simulink model "quater_car"  (R2025b)
settings: Solver=FixedStepAuto  StartTime=0.0  StopTime=10.0  FixedStep=0.001  RelTol=1e-3
values from neighbouring files (symbols this model uses):
  cs = cs_n(n)    [sim2.m]    (also in sim2_part2.m = 50)
  cs_nolinear = i    [sim2_part2.m]
  ct = 0.01 * 12    (= 0.12)    [sim2.m]    (also in sim2_part2.m)
  ks = 100 * 12    (= 1200)    [sim2.m]    (also in sim2_part2.m)
  kt = 1000 * 12    (= 12000)    [sim2.m]    (also in sim2_part2.m)
  ms = Ws/g    (= 83.9291265154)    [Final_sim.m]    (also in Final_sim_nonlinear.m; sim2.m = 31.0848616724; sim2_part2.m = 31.0848616724)
  mu = 100/32.17    (= 3.10848616724)    [sim2.m]    (also in sim2_part2.m)
  Road_type = 6    [sim2_part2.m]
libraries: dspsrcs4 x1
settings Model: Creator=elijah  LastModifiedBy=elijah

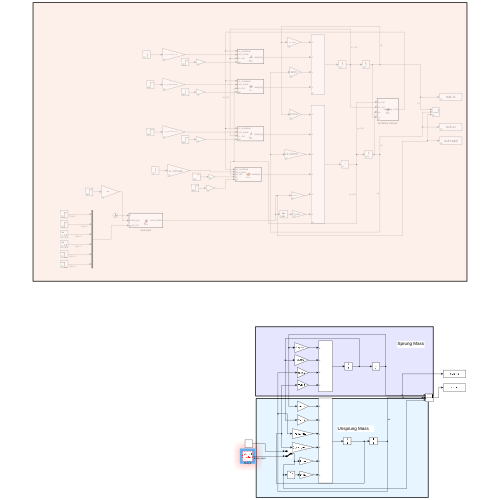
[thumbnail: Simulink's stored preview of the top-level diagram]
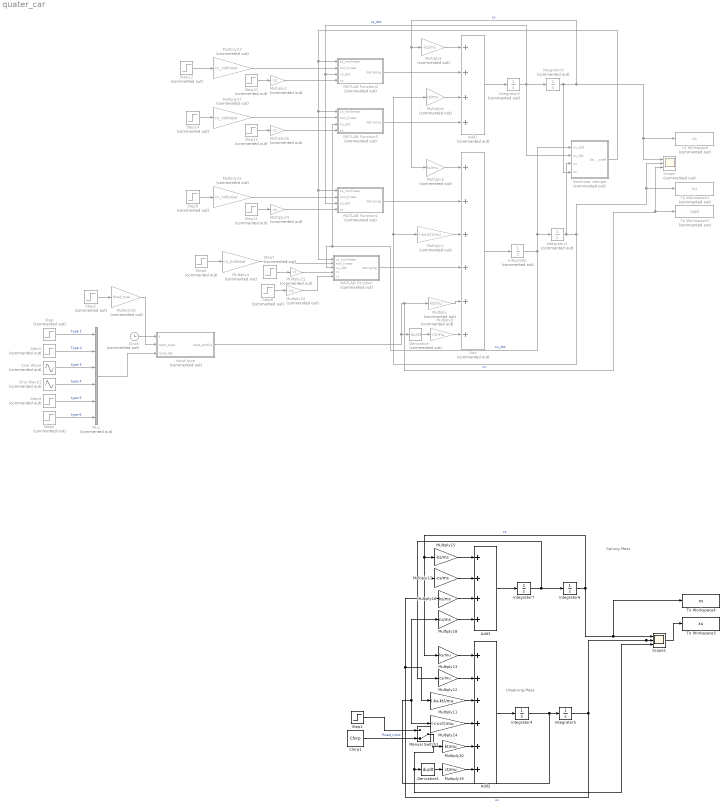
== system quater_car ==
  note: Sprung Mass
  note: Unsprung Mass
  Add : Sum  Commented=on  Inputs=++++++
  Add1 : Sum  Commented=on  Inputs=++++
  Add2 : Sum  Inputs=++++++
  Add3 : Sum  Inputs=++++
  Chirp1 : dspsrcs4/Chirp  sweep=Linear  mode=Unidirectional  f0=0  f1=12  t1=100  Tsweep=100  phase=0  Ts=1/1000  spf=1  datatype=double  OutputFrames=off
  Clock : Clock  Commented=on
  Derivative : Derivative  Commented=on
  Derivative1 : Derivative
  Input type : MATLAB Function  Commented=on  TreatAsAtomicUnit=on
  Integrator{,1..3} (4 alike) : Integrator  Commented=on
  Integrator{4..7} (4 alike) : Integrator
  MATLAB Function : MATLAB Function  Commented=on  TreatAsAtomicUnit=on
  MATLAB Function1 : MATLAB Function  Commented=on  TreatAsAtomicUnit=on
  MATLAB Function2 : MATLAB Function  Commented=on  TreatAsAtomicUnit=on
  MATLAB Function3 : MATLAB Function  Commented=on  TreatAsAtomicUnit=on
  Manual Switch1 : ManualSwitch  CurrentSetting=0
  Multiply : Gain  Commented=on  Gain=kt/mu
  Multiply1 : Gain  Commented=on  Gain=(-ks-kt)/mu
  Multiply10 : Gain  Gain=kt/mu
  Multiply11 : Gain  Gain=(-ks-kt)/mu
  Multiply12 : Gain  Gain=cs/mu
  Multiply13 : Gain  Gain=ks/mu
  Multiply14 : Gain  Gain=(-cs-ct)/mu
  Multiply15 : Gain  Gain=-ks/ms
  Multiply16 : Gain  Gain=ks/ms
  Multiply17 : Gain  Gain=-cs/ms
  Multiply18 : Gain  Gain=cs/ms
  Multiply19 : Gain  Gain=ct/mu
  Multiply{2,22,24,26} (4 alike) : Gain  Commented=on  Gain=cs
  Multiply20 : Gain  Commented=on  Gain=Road_type
  Multiply21 : Gain  Commented=on  Gain=ct
  Multiply{4,23,25,27} (4 alike) : Gain  Commented=on  Gain=cs_nolinear
  Multiply3 : Gain  Commented=on  Gain=ks/mu
  Multiply5 : Gain  Commented=on  Gain=-ks/ms
  Multiply6 : Gain  Commented=on  Gain=ks/ms
  Multiply9 : Gain  Commented=on  Gain=ct/mu
  Mux : Mux  Commented=on  Inputs=6
  Nonlinear damper : MATLAB Function  Commented=on  TreatAsAtomicUnit=on
  Scope : Scope  Commented=on  NumInputPorts=3
      settings: ActiveDisplayYMinimum=-0.37333179506609859  ActiveDisplayYMaximum=0.29861915376867731
  Scope1 : Scope  NumInputPorts=3
      settings: ActiveDisplayYMinimum=0.90310451552336024  ActiveDisplayYMaximum=1.0409550070632758
  Sine Wave : Sin  Commented=on  Amplitude=0.083333  Frequency=6.283185  SampleTime=0
  Sine Wave1 : Sin  Commented=on  Amplitude=0.02083333  Frequency=62.8318  SampleTime=0
  Step : Step  Commented=on  Time=2  After=0.08333  SampleTime=2
  Step1 : Step  Time=5  SampleTime=0
  Step{2,6..14} (10 alike) : Step  Commented=on  Time=0  SampleTime=0
  Step3 : Step  Commented=on  Time=2  After=0.0208333  SampleTime=2
  Step4 : Step  Commented=on  Time=0  After=-0.1666667  SampleTime=1
  Step5 : Step  Commented=on  Time=2  After=-0.1666667  SampleTime=1
  To Workspace : ToWorkspace  Commented=on  VariableName=xs  SaveFormat=Timeseries  SampleTime=-1
  To Workspace1 : ToWorkspace  Commented=on  VariableName=xu  SaveFormat=Timeseries  SampleTime=-1
  To Workspace2 : ToWorkspace  Commented=on  VariableName=road  SaveFormat=Timeseries  SampleTime=-1
  To Workspace3 : ToWorkspace  VariableName=xu  SaveFormat=Timeseries  SampleTime=-1
  To Workspace4 : ToWorkspace  VariableName=xs  SaveFormat=Timeseries  SampleTime=-1
  wires:
  Multiply1/1 -> Add/3
  MATLAB Function1/1(damping) -> Add/2
  Multiply3/1 -> Add/1
  Integrator/1 -> Nonlinear damper/1(xu_dot), Integrator1/1, MATLAB Function3/3(xu_dot), MATLAB Function/3(xu_dot)  "xu_dot"
  Add/1 -> Integrator/1
  Integrator1/1 -> Nonlinear damper/3(xu), Multiply6/1, Multiply1/1, Scope/2, To Workspace1/1  "xu"
  Multiply5/1 -> Add1/1
  Multiply6/1 -> Add1/3
  MATLAB Function2/1(damping) -> Add1/2
  Integrator3/1 -> Multiply3/1, Multiply5/1, Scope/1, To Workspace/1, Nonlinear damper/4(xs)  "xs"
  Add1/1 -> Integrator2/1
  Integrator2/1 -> Nonlinear damper/2(xs_dot), MATLAB Function1/3(xs_dot), MATLAB Function2/3(xs_dot), Integrator3/1  "xs_dot"
  Multiply/1 -> Add/5
  Multiply9/1 -> Add/6
  Derivative/1 -> Multiply9/1
  Step/1 -> Mux/1  "Type 1"
  Manual Switch1/1 -> Scope1/3, Derivative1/1, Multiply10/1
  Step1/1 -> Manual Switch1/1
  Derivative1/1 -> Multiply19/1
  Multiply19/1 -> Add2/6
  Add3/1 -> Integrator7/1
  Multiply12/1 -> Add2/2
  Multiply16/1 -> Add3/3
  Multiply17/1 -> Add3/2
  Integrator6/1 -> Multiply13/1, Multiply15/1, To Workspace4/1, Scope1/1  "xs"
  Multiply18/1 -> Add3/4
  Integrator7/1 -> Integrator6/1, Multiply12/1, Multiply17/1
  Chirp1/1 -> Manual Switch1/2  "Road_input"
  Multiply15/1 -> Add3/1
  Multiply11/1 -> Add2/3
  Multiply13/1 -> Add2/1
  Multiply14/1 -> Add2/4
  Integrator4/1 -> Integrator5/1, Multiply18/1, Multiply14/1
  Add2/1 -> Integrator4/1
  Integrator5/1 -> To Workspace3/1, Scope1/2, Multiply16/1, Multiply11/1  "ux"
  Multiply10/1 -> Add2/5
  Mux/1 -> Input type/3(road_set)
  Input type/1(road_profile) -> To Workspace2/1, Scope/3, Multiply/1, Derivative/1
  Multiply20/1 -> Input type/2(road_type)
  Step2/1 -> Multiply20/1
  Step3/1 -> Mux/2  "Type 2"
  Sine Wave/1 -> Mux/3  "type 3"
  Sine Wave1/1 -> Mux/4  "type 4"
  Step4/1 -> Mux/5  "type 5"
  Step5/1 -> Mux/6  "type 6"
  Clock/1 -> Input type/1(t)
  MATLAB Function/1(damping) -> Add/4
  Multiply4/1 -> MATLAB Function/2(non_linear)
  Step6/1 -> Multiply4/1
  Multiply21/1 -> MATLAB Function/4(ct)
  Step7/1 -> Multiply21/1
  Step8/1 -> Multiply22/1
  Multiply22/1 -> MATLAB Function/5(cs)
  Nonlinear damper/1(damping_coef) -> MATLAB Function2/1(cs_nonlinear), MATLAB Function3/1(cs_nonlinear), MATLAB Function1/1(cs_nonlinear), MATLAB Function/1(cs_nonlinear)
  Multiply25/1 -> MATLAB Function1/2(non_linear)
  Step11/1 -> Multiply24/1
  Multiply24/1 -> MATLAB Function1/4(cs)
  Step9/1 -> Multiply25/1
  Multiply2/1 -> MATLAB Function2/4(cs)
  Step12/1 -> Multiply23/1
  Step10/1 -> Multiply2/1
  Multiply23/1 -> MATLAB Function2/2(non_linear)
  Multiply27/1 -> MATLAB Function3/2(non_linear)
  Step13/1 -> Multiply26/1
  Step14/1 -> Multiply27/1
  Multiply26/1 -> MATLAB Function3/4(cs)
  MATLAB Function3/1(damping) -> Add1/4

== matlab function quater_car/Input type ==
  data: t input; road_type input; road_set input; road_profile output
function road_profile = fcn(t, road_type, road_set)

int = road_type(1,1);


if int == 5
    if (2<=t)&&(t<=2.03409)
        road_profile = road_set(int,:);
    else
        road_profile = road_set(int,:)*0;
    end
elseif int == 6
    if (2<=t)&&(t<=2.06818)
        road_profile = road_set(int,:);
    else
        road_profile = road_set(int,:)*0;
    end

else
    road_profile = road_set(int,:);
end

== matlab function quater_car/MATLAB Function ==
  data: cs_nonlinear input; non_linear input; xu_dot input; damping output; ct input; cs input
function damping = fcn(cs_nonlinear, non_linear, xu_dot, ct, cs)
mu =100/32.17;
if non_linear ==1
    damping = ((-ct-cs_nonlinear)/(mu))*xu_dot;
else
    damping = ((-ct-cs)/(mu))*xu_dot;
end

== matlab function quater_car/Nonlinear damper ==
  data: xu_dot input; xs_dot input; damping_coef output; xu input; xs input
function damping_coef = fcn(xu_dot, xs_dot, xu, xs)

xrel = xu-xs;
dxrel = xu_dot-xs_dot;


%% sky hook nonlinear damping
%if dxrel>=0
 %   C = 30;
%else
%    C = 1;
%end



%% non linear damping made up expose
C = 30*exp(xrel*30) + 20*exp(-dxrel*2) + 30; % trahs when not a setp input

%%

C = 30/(1*dxrel + 1) + 30 - 1*(dxrel); %% aplified when out of phase
if C>1000
   C = 30;
end


%% 

if xrel >0 

    C = 5*dxrel.^2 + 50;
else 
    C = 5*dxrel.^2 - 50;
end


%% sky hook 


if xs_dot*(dxrel) <0 

    C = 50;
else 
    C = 10;
end


damping_coef = C;

== matlab function quater_car/MATLAB Function1 ==
  data: cs_nonlinear input; non_linear input; xs_dot input; damping output; cs input
function damping = fcn(cs_nonlinear, non_linear, xs_dot, cs)
mu =100/32.17;
if non_linear ==1
    damping = ((cs_nonlinear)/(mu))*xs_dot;
else
    damping = ((cs)/(mu))*xs_dot;
end

== matlab function quater_car/MATLAB Function2 ==
  data: cs_nonlinear input; non_linear input; xs_dot input; damping output; cs input
function damping = fcn(cs_nonlinear, non_linear, xs_dot, cs)
ms =1000/32.17;
if non_linear ==1
    damping = ((-cs_nonlinear)/(ms))*xs_dot;
else
    damping = ((-cs)/(ms))*xs_dot;
end

== matlab function quater_car/MATLAB Function3 ==
  data: cs_nonlinear input; non_linear input; xu_dot input; damping output; cs input
function damping = fcn(cs_nonlinear, non_linear, xu_dot, cs)
ms =1000/32.17;
if non_linear ==1
    damping = ((cs_nonlinear)/(ms))*xu_dot;
else
    damping = ((cs)/(ms))*xu_dot;
end
